simulink library "pmm"  (R2021b)
settings: Solver=VariableStepAuto  StartTime=0.0  StopTime=10.0  RelTol=1e-3
undefined symbols (not defined in the file): APMM_CoolgFanActCurr_X_pct, APMM_EWP1Curr_X_c, APMM_EWP3Curr_X_c, APMM_LVBattChktime_X_enum, APMM_LVBattChrgtime_X_enum, APMM_LVChrgLv_X_mV, ENUM_ANTITHEFT_ALARM, ENUM_ANTITHEFT_ARM, ENUM_ANTITHEFT_DISARM, ENUM_ANTITHEFT_WAIT, ENUM_APSSYSTEMSTA_REMOTEACTIVE, ENUM_CHRGPLUGSTA_NONE, ENUM_CRASHSTATE_FRONTFIRSTLV, ENUM_CRASHSTATE_LEFTSIDE, ENUM_CRASHSTATE_RIGHTSIDE, ENUM_DRIVETRAIN_AWD, ENUM_DRIVETRAIN_FWD, ENUM_DRIVETRAIN_RWD, ENUM_DRSEATSTA_EMPTY, ENUM_DRSEATSTA_INVALID, ENUM_DRSEATSTA_OCCUPIED, ENUM_EPBSTA_APPLIED, ENUM_GEARACTUALPOSN_D, ENUM_GEARACTUALPOSN_N, ENUM_GEARACTUALPOSN_P, ENUM_GEARACTUALPOSN_R, ENUM_HVBATTREADYPRE_READY, ENUM_OTACHKSTA_NOREQUEST, ENUM_OTACHKSTA_NOTIMEOUT, ENUM_OTACHKSTA_TIMEOUT, ENUM_PDKEYRAWLULOCK_INLOCK, ENUM_PDKEYRAWLULOCK_INUNLOCK, ENUM_PDKEYRAWPS_INPS, ENUM_PDKEYSTA_LOCK, ENUM_PDKEYSTA_PS, ENUM_PDKEYSTA_UNAVALIABLE, ENUM_PDKEYSTA_UNLOCK, ENUM_POWERSTA_OFF, ENUM_POWERSTA_OFFC, ENUM_POWERSTA_STANDBY, ENUM_PWRREQOTA_NOREQUEST, ENUM_PWRREQOTA_REQPOWEROFF, ENUM_PWRREQOTA_REQPOWERSTDBY, ENUM_PWRSTASW_READY, ENUM_V2LSTA_NOPLUG, ENUM_VEHICLETYPE_D31L24, ENUM_VEHMALFUNLEVEL_LEVEL3, ENUM_VEHMALFUNLEVEL_LEVEL4, FALSE, KPMM_AllDoorClosedHoldTime_s, KPMM_APSAllowThd_pct, KPMM_BattDownFailtime_s, KPMM_BattUpFailtime_s, KPMM_BattUpResetRty_cnt, KPMM_BattUpResetSW_flg, KPMM_BattUpResetTO_s, KPMM_BattUpRstDlyTO_s, KPMM_BrakeSWHoldTime_s, KPMM_CANValidChkFailtime_s, KPMM_ChrgPlugHoldTime_s ... (+87)
libraries: simulink x29, hcu_lib x24
(part 5 of 7)

== stateflow chart pmm/PMM/PMM/RequirementManagementForPowerUp ==
  state RequirementManagementForPowerUp
    note: [VINP_HVBattSOC_pct <= KPMM_HVBattSOCPwrDwnThd_pct]
    (default) -> (junction 135)
    RequirementManagementForPowerUp -> (junction 135) [order 2]
    (junction 135) -> (junction 3) : {VPMM_PwrUpReq_enum = ENUM_PWRUPREQ_NOREQUEST;
        |  VPMM_PwrStaSelect_enum = ENUM_PWRSTASELECT_NOREQUEST;}
    (junction 3) -> (junction 158) [order 1] : [(VPMM_PowerSta_enum == ENUM_POWERSTA_OFF || ...
        |   VPMM_PowerSta_enum == ENUM_POWERSTA_STANDBY) && ...
        |  VPMM_OTAPwrReqOFFChkSta_enum != ENUM_OTACHKSTA_NOTIMEOUT && ...
        |  VPMM_OTAPwrReqStdChkSta_enum != ENUM_OTACHKSTA_NOTIMEOUT]
    (junction 158) -> (junction 5) [order 1] : [(VPMM_DetectDoorOpened_flg || ...
        |   VPMM_BrkPedalRisingEdge_flg || ...
        |   (VPMM_BrkPedalPressed_flg && VPMM_PreOFF_flg)) && ...
        |  VPMM_PowerSta_enum == ENUM_POWERSTA_STANDBY]
        | {VPMM_PwrStaSelect_enum = ENUM_PWRSTASELECT_GOON;}
    (junction 3) -> (junction 6) [order 2]
    (junction 158) -> (junction 162) [order 2]
    (junction 5) -> (junction 8)
    (junction 8) -> (junction 167) [order 1] : [VPMM_PowerUpState_enum == ENUM_PUSTATE_POWERUPFAIL]
    (junction 8) -> (junction 169) [order 2] : {VPMM_PwrUpReq_enum = ENUM_PWRUPREQ_USERREQPU;}
    (junction 167) -> (junction 171)
    (junction 162) -> (junction 164) [order 1] : [(VPMM_ChrgPlugInRisingEdge_flg && VPMM_PowerSta_enum == ENUM_POWERSTA_STANDBY)|| ...
        |  (VPMM_LVSilentChrgReqStd_flg && ((!VINP_HoodSW_flg) || (VPMM_Delay4IVIWarnAct_flg))) || ...
        |  VPMM_LVSilentChrgReq_flg || ...
        |  (VINP_EvccAplusPwrUpReq_flg && VINP_ChrgPlugSta_enum != ENUM_CHRGPLUGSTA_NONE)]
        | {VPMM_PwrStaSelect_enum = ENUM_PWRSTASELECT_GOOFFC;}
    (junction 164) -> (junction 173) [order 1] : [VTQD_GearActualPosn_enum == ENUM_GEARACTUALPOSN_P && ...
        |  VINP_VehSpeed_kph < KPMM_PwrUpVehSpdThd_kph]
    (junction 162) -> (junction 237) [order 2]
    (junction 164) -> (junction 225) [order 2]
    (junction 173) -> (junction 239)
    (junction 237) -> (junction 239) [order 1] : [(VINP_PwrReq_OTA_enum == ENUM_PWRREQOTA_REQPOWERON && VINP_HVBattSOC_pct > KPMM_HVBattSOCPwrDwnThd_pct) || ...
        | (VINP_APSPwrReq_enum == ENUM_PWRREQPAPS_REQPWRREADY && VPMM_PwrReqRAPSAvail_flg)]
        | {VPMM_PwrStaSelect_enum = ENUM_PWRSTASELECT_GOON;}
    (junction 237) -> (junction 242) [order 2]
    (junction 239) -> (junction 244)
    (junction 242) -> (junction 244) [order 1] : [(VINP_SchedChgwake_flg == ENUM_SCHEDCHG_WAKE && ...
        |   VINP_ChrgPlugSta_enum != ENUM_CHRGPLUGSTA_NONE)]
        | {VPMM_PwrStaSelect_enum = ENUM_PWRSTASELECT_GOOFFC;}
    (junction 242) -> (junction 248) [order 2]
    (junction 244) -> (junction 250)
    (junction 248) -> (junction 250) [order 1] : [VINP_HVBPreheatPrecoolSta_enum == ENUM_HVBPRESTA_PREHEAT || ...
        |  VINP_HVBPreheatPrecoolSta_enum == ENUM_HVBPRESTA_PRECOOL]
        | {VPMM_PwrStaSelect_enum = ENUM_PWRSTASELECT_GOOFFA;}
    (junction 248) -> (junction 179) [order 2]
    (junction 250) -> (junction 194)
    (junction 179) -> (junction 181) [order 1] : [VINP_RePwrReqTbox_enum == ENUM_REPWRREQTBOX_REQVEHCHK || ...
        |  VINP_RePwrReqTbox_enum == ENUM_REPWRREQTBOX_REQDTC || ...
        |  VINP_RePwrReqTbox_enum == ENUM_REPWRREQTBOX_REQRADIO || ...
        |  VINP_RePwrReqTbox_enum == ENUM_REPWRREQTBOX_REQON || ...
        |  VINP_RePwrReqDKCT_enum == ENUM_REPWRREQDKC_REQVEHCHK || ...
        |  VINP_RePwrReqDKCT_enum == ENUM_REPWRREQDKC_REQDTC || ...
        |  VINP_RePwrReqDKCT_enum == ENUM_REPWRREQDKC_REQRADIO || ...
        |  VINP_RePwrReqDKCT_enum == ENUM_REPWRREQDKC_REQON]
        | {VPMM_PwrStaSelect_enum = ENUM_PWRSTASELECT_GOON;}
    (junction 179) -> (junction 183) [order 2]
    (junction 181) -> (junction 185)
    (junction 183) -> (junction 185) [order 1] : [VINP_RePwrReqTbox_enum == ENUM_REPWRREQTBOX_REQACTEMP || ...
        |  VINP_RePwrReqDKCT_enum == ENUM_REPWRREQDKC_REQACTEMP]
        | {VPMM_PwrStaSelect_enum = ENUM_PWRSTASELECT_GOOFFA;}
    (junction 183) -> (junction 190) [order 2]
    (junction 185) -> (junction 9)
    (junction 9) -> (junction 194) [order 1] : [VTQD_GearActualPosn_enum == ENUM_GEARACTUALPOSN_P && ...
        |  !VPMM_BMSWarn_flg && ...
        |  VINP_VehSpeed_kph < 2 && ...
        |  VINP_HVBattSOC_pct > KPMM_HVBattSOCPwrDwnThd_pct && ...
        |  VPMM_AllDoorClosed_flg && ...
        |  !VINP_HoodSW_flg && ...
        |  !VINP_TailgateSW_flg && ...
        |  VBCM_AntitheftSta_enum == ENUM_ANTITHEFT_ARM]
        | {VPMM_ReVehThdChkSta_enum = ENUM_REVEHSTA_CHECKOK;}
    (junction 194) -> (junction 197) [order 1] : [VPMM_PowerUpState_enum == ENUM_PUSTATE_POWERUPFAIL]
    (junction 9) -> (junction 11) [order 2]
    (junction 194) -> (junction 204) [order 2] : {VPMM_PwrUpReq_enum = ENUM_PWRUPREQ_SYSREQPU;}
    (junction 197) -> (junction 200)
    (junction 11) -> (junction 12) [order 1] : [VTQD_GearActualPosn_enum != ENUM_GEARACTUALPOSN_P]
        | {VPMM_ReVehThdChkSta_enum = ENUM_REVEHSTA_GEARPOSITIONERROR;}
    (junction 11) -> (junction 15) [order 2]
    (junction 15) -> (junction 16) [order 1] : [VPMM_BMSWarn_flg]
        | {VPMM_ReVehThdChkSta_enum = ENUM_REVEHSTA_HVBERR;}
    (junction 15) -> (junction 17) [order 2]
    (junction 17) -> (junction 18) [order 1] : [VINP_VehSpeed_kph >= 2]
        | {VPMM_ReVehThdChkSta_enum = ENUM_REVEHSTA_VEHNOTSTEADYSTATE;}
    (junction 17) -> (junction 21) [order 2]
    (junction 21) -> (junction 22) [order 1] : [VBCM_AntitheftSta_enum != ENUM_ANTITHEFT_ARM]
        | {VPMM_ReVehThdChkSta_enum = ENUM_REVEHSTA_ANTITHEFTNOTARM;}
    (junction 21) -> (junction 26) [order 2]
    (junction 26) -> (junction 27) [order 1] : [!VPMM_AllDoorClosed_flg || ...
        |  VINP_HoodSW_flg || ...
        |  VINP_TailgateSW_flg]
        | {VPMM_ReVehThdChkSta_enum = ENUM_REVEHSTA_ANYDOOROPEN;}
    (junction 26) -> (junction 29) [order 2]
    (junction 29) -> (junction 30) : {VPMM_ReVehThdChkSta_enum = ENUM_REVEHSTA_HVBSOCLOW;}
    (junction 29) -> (junction 31) [commented out] : {VPMM_ReVehThdChkSta_enum = ENUM_REVEHSTA_CHECKINVALID;}
    (junction 169) -> (junction 204)
    (junction 204) -> (junction 32)
    RequirementManagementForPowerUp -> (junction 32) [order 1] : [VPMM_PwrUpChk_flg]
        | {VPMM_PwrUpChk_flg = FALSE;}
    (junction 32) -> (junction 139) [order 1] : [VPMM_PowerUpState_enum == ENUM_PUSTATE_COMPLETED]
        | {VPMM_PwrUpChkFailtimer_s = 0;}
    (junction 32) -> (junction 141) [order 2]
    (junction 141) -> (junction 143) [order 1] : [VPMM_PwrUpChkFailtimer_s >= KPMM_PwrUpChkFailtime_s]
        | {VPMM_PwrUpChkFailtimer_s = 0;}
    (junction 141) -> (junction 145) [order 2] : {VPMM_PwrUpChk_flg = TRUE;
        |  VPMM_PwrUpChkFailtimer_s += task_time_s;}
  data: task_time_s input; VINP_HVBPreheatPrecoolSta_enum input; VINP_HVBattSOC_pct input; VINP_HoodSW_flg input; VINP_TailgateSW_flg input; VINP_SchedChgwake_flg input; VINP_VehSpeed_kph input; VPMM_AllDoorClosed_flg input; VBCM_AntitheftSta_enum input; VPMM_BMSWarn_flg input; VPMM_BrkPedalPressed_flg input; VPMM_BrkPedalRisingEdge_flg input; VPMM_ChrgPlugInRisingEdge_flg input; VPMM_DetectDoorOpened_flg input; VPMM_LVSilentChrgReq_flg input boolean; VPMM_PowerSta_enum input uint8; VTQD_GearActualPosn_enum input; VINP_PwrReq_OTA_enum input; VINP_RePwrReqDKCT_enum input; VINP_RePwrReqTbox_enum input; VPMM_PwrStaSelect_enum output; VPMM_PwrUpReq_enum output; VPMM_ReVehThdChkSta_enum output; ENUM_ANTITHEFT_ARM parameter; ENUM_GEARACTUALPOSN_P parameter; ENUM_HVBPRESTA_PRECOOL parameter; ENUM_HVBPRESTA_PREHEAT parameter; ENUM_POWERSTA_OFF parameter; ENUM_POWERSTA_STANDBY parameter; ENUM_PWRREQOTA_REQPOWERON parameter; ENUM_PWRSTASELECT_GOOFFA parameter; ENUM_PWRSTASELECT_GOOFFC parameter; ENUM_PWRSTASELECT_GOON parameter; ENUM_PWRSTASELECT_NOREQUEST parameter; ENUM_PWRUPREQ_NOREQUEST parameter; ENUM_PWRUPREQ_SYSREQPU parameter; ENUM_PWRUPREQ_USERREQPU parameter; ENUM_REPWRREQDKC_REQACTEMP parameter; ENUM_REPWRREQDKC_REQDTC parameter; ENUM_REPWRREQDKC_REQON parameter; ENUM_REPWRREQDKC_REQRADIO parameter; ENUM_REPWRREQDKC_REQVEHCHK parameter; ENUM_REPWRREQTBOX_REQACTEMP parameter; ENUM_REPWRREQTBOX_REQDTC parameter; ENUM_REPWRREQTBOX_REQON parameter; ENUM_REPWRREQTBOX_REQRADIO parameter; ENUM_REPWRREQTBOX_REQVEHCHK parameter; ENUM_REVEHSTA_ANTITHEFTNOTARM parameter; ENUM_REVEHSTA_ANYDOOROPEN parameter; ENUM_REVEHSTA_CHECKINVALID parameter; ENUM_REVEHSTA_CHECKOK parameter; ENUM_REVEHSTA_GEARPOSITIONERROR parameter; ENUM_REVEHSTA_HVBERR parameter; ENUM_REVEHSTA_HVBSOCLOW parameter; ENUM_REVEHSTA_VEHNOTSTEADYSTATE parameter; ENUM_SCHEDCHG_WAKE parameter; VPMM_PowerUpState_enum input uint8; VPMM_PwrUpChkFailtimer_s local single; VPMM_PwrUpChk_flg local boolean; ENUM_PUSTATE_COMPLETED parameter; FALSE parameter; TRUE parameter; VINP_ChrgPlugSta_enum input uint8; VINP_EvccAplusPwrUpReq_flg input boolean; VPMM_LVSilentChrgReqStd_flg input boolean; ENUM_PUSTATE_POWERUPFAIL parameter; VPMM_PreOFF_flg input boolean; ENUM_CHRGPLUGSTA_NONE parameter; VPMM_OTAPwrReqOFFChkSta_enum input uint8; VPMM_OTAPwrReqStdChkSta_enum input uint8; ENUM_OTACHKSTA_NOTIMEOUT parameter; KPMM_HVBattSOCPwrDwnThd_pct input; VINP_APSPwrReq_enum input uint8; VPMM_PwrReqRAPSAvail_flg input boolean; ENUM_PWRREQPAPS_REQPWRREADY parameter; KPMM_PwrUpChkFailtime_s input; VPMM_Delay4IVIWarnAct_flg input; KPMM_PwrUpVehSpdThd_kph input

== stateflow chart pmm/PMM/PMM/RequirementManagementForPowerStateConstrain ==
  state RequirementManagementForPowerStateConstrain
    (default) -> (junction 2) : {VPMM_TCountSta_enum = ENUM_TCOUNTSTA_NOCOUNTING;
        |  VPMM_PwrOffTimer_s = 0;}
    RequirementManagementForPowerStateConstrain -> (junction 2) [order 2]
    (junction 2) -> (junction 3) : {VPMM_PwrStaConstraint_enum = ENUM_PWRCONSTRAINT_NOREQUEST;}
    RequirementManagementForPowerStateConstrain -> (junction 3) [order 1] : [VPMM_ConstraintLoop_flg]
        | {VPMM_ConstraintLoop_flg = FALSE;}
    (junction 3) -> (junction 4) [order 1] : [VPMM_PowerSta_enum == ENUM_POWERSTA_ON || ...
        |  VPMM_PowerSta_enum == ENUM_POWERSTA_OFFA || ...
        |  VPMM_PowerSta_enum == ENUM_POWERSTA_OFFC]
    (junction 4) -> (junction 5) [order 1] : [VINP_PwrReq_OTA_enum == ENUM_PWRREQOTA_REQPOWERON || ...
        |  VINP_OFFACMODE_enum == ENUM_OFFACMODE_CAMP]
    (junction 3) -> (junction 6) [order 2]
    (junction 4) -> (junction 7) [order 2]
    (junction 5) -> (junction 8) : {VPMM_PwrStaConstraint_enum = ENUM_PWRCONSTRAINT_PWRSTAON;}
    (junction 7) -> (junction 8) [order 1] : [VINP_AVMOFFRecButt_flg == ENUM_AVMOFFRECBUTT_ON || ...
        |  VINP_OFFACMODE_enum == ENUM_OFFACMODE_PET || ...
        |  VINP_OFFACMODE_enum == ENUM_OFFACMODE_ON || ...
        |  VINP_HVBPreheatPrecoolSta_enum == ENUM_HVBPRESTA_PREHEAT || ...
        |  VINP_HVBPreheatPrecoolSta_enum == ENUM_HVBPRESTA_PRECOOL]
        | {VPMM_PwrStaConstraint_enum = ENUM_PWRCONSTRAINT_HVACTIVE;}
    (junction 7) -> (junction 80) [order 2]
    (junction 8) -> (junction 9) : {VPMM_TCountSta_enum = ENUM_TCOUNTSTA_NOCOUNTING;
        |  VPMM_PwrOffTimer_s = 0;
        |  VPMM_ConstraintLoop_flg = TRUE;}
    (junction 80) -> (junction 82) [order 1] : [VPMM_TCountSta_enum == ENUM_TCOUNTSTA_COUNTINGFINISH]
    (junction 82) -> (junction 90) [order 1] : [VPMM_PwrStaSW_enum == ENUM_PWRSTASW_PWRDOWN]
    (junction 80) -> (junction 10) [order 2]
    (junction 82) -> (junction 84) [order 2]
    (junction 90) -> (junction 92) : {VPMM_TCountSta_enum = ENUM_TCOUNTSTA_NOCOUNTING;}
    (junction 10) -> (junction 11) [order 1] : [(VPMM_PowerOffTSet_s > 0 && ...
        |   (VINP_RePwrReqTbox_enum == ENUM_REPWRREQTBOX_REQVEHCHK || ...
        |    VINP_RePwrReqTbox_enum == ENUM_REPWRREQTBOX_REQDTC || ...
        |    VINP_RePwrReqTbox_enum == ENUM_REPWRREQTBOX_REQRADIO || ...
        |    VINP_RePwrReqTbox_enum == ENUM_REPWRREQTBOX_REQON)) || ...
        |  (VPMM_PowerOffTSetDKC_enum > 0 && ...
        |   (VINP_RePwrReqDKCT_enum == ENUM_REPWRREQDKC_REQVEHCHK || ...
        |    VINP_RePwrReqDKCT_enum == ENUM_REPWRREQDKC_REQDTC || ...
        |    VINP_RePwrReqDKCT_enum == ENUM_REPWRREQDKC_REQRADIO || ...
        |    VINP_RePwrReqDKCT_enum == ENUM_REPWRREQDKC_REQON))]
    (junction 10) -> (junction 12) [order 2]
    (junction 11) -> (junction 13) : {VPMM_PwrStaConstraint_enum = ENUM_PWRCONSTRAINT_ONFORTIME;}
    (junction 12) -> (junction 13) [order 1] : [(VPMM_PowerOffTSet_s > 0 && ...
        |   VINP_RePwrReqTbox_enum == ENUM_REPWRREQTBOX_REQACTEMP) || ...
        |  (VPMM_PowerOffTSetDKC_enum > 0 && ...
        |   VINP_RePwrReqDKCT_enum == ENUM_REPWRREQDKC_REQACTEMP)]
        | {VPMM_PwrStaConstraint_enum = ENUM_PWRCONSTRAINT_HVFORTIME;}
    (junction 13) -> (junction 14) [order 1] : [(VPMM_PowerOffTSet_s >= VPMM_PowerOffTSetDKC_enum && VPMM_PwrOffTimer_s >= VPMM_PowerOffTSet_s) || ...
        |  (VPMM_PowerOffTSetDKC_enum > VPMM_PowerOffTSet_s && VPMM_PwrOffTimer_s >= VPMM_PowerOffTSetDKC_enum)]
    (junction 12) -> (junction 15) [order 2] : {VPMM_TCountSta_enum = ENUM_TCOUNTSTA_NOCOUNTING;
        |  VPMM_PwrOffTimer_s = 0;}
    (junction 13) -> (junction 16) [order 2] : {VPMM_TCountSta_enum = ENUM_TCOUNTSTA_TIMMERCOUNTING;
        |  VPMM_PwrOffTimer_s += task_time_s;
        |  VPMM_ConstraintLoop_flg = TRUE;}
    (junction 14) -> (junction 17) : {VPMM_TCountSta_enum = ENUM_TCOUNTSTA_COUNTINGFINISH;
        |  VPMM_PwrStaConstraint_enum = ENUM_PWRCONSTRAINT_NOREQUEST;
        |  VPMM_PwrOffTimer_s = 0;}
  data: task_time_s input; VPMM_PowerSta_enum input; VINP_AVMOFFRecButt_flg input; VINP_HVBPreheatPrecoolSta_enum input; VINP_OFFACMODE_enum input; VPMM_PowerOffTSet_s input; VPMM_PowerOffTSetDKC_enum input; VINP_PwrReq_OTA_enum input; VINP_RePwrReqDKCT_enum input; VINP_RePwrReqTbox_enum input; VPMM_PwrStaConstraint_enum output; VPMM_TCountSta_enum output; VPMM_PwrOffTimer_s local single; ENUM_AVMOFFRECBUTT_ON parameter; ENUM_HVBPRESTA_PRECOOL parameter; ENUM_HVBPRESTA_PREHEAT parameter; ENUM_OFFACMODE_CAMP parameter; ENUM_OFFACMODE_ON parameter; ENUM_OFFACMODE_PET parameter; ENUM_POWERSTA_OFFA parameter; ENUM_POWERSTA_OFFC parameter; ENUM_POWERSTA_ON parameter; ENUM_PWRCONSTRAINT_HVACTIVE parameter; ENUM_PWRCONSTRAINT_HVFORTIME parameter; ENUM_PWRCONSTRAINT_NOREQUEST parameter; ENUM_PWRCONSTRAINT_ONFORTIME parameter; ENUM_PWRCONSTRAINT_PWRSTAON parameter; ENUM_PWRREQOTA_REQPOWERON parameter; ENUM_REPWRREQDKC_REQACTEMP parameter; ENUM_REPWRREQDKC_REQDTC parameter; ENUM_REPWRREQDKC_REQON parameter; ENUM_REPWRREQDKC_REQRADIO parameter; ENUM_REPWRREQDKC_REQVEHCHK parameter; ENUM_REPWRREQTBOX_REQACTEMP parameter; ENUM_REPWRREQTBOX_REQDTC parameter; ENUM_REPWRREQTBOX_REQON parameter; ENUM_REPWRREQTBOX_REQRADIO parameter; ENUM_REPWRREQTBOX_REQVEHCHK parameter; ENUM_TCOUNTSTA_COUNTINGFINISH parameter; ENUM_TCOUNTSTA_NOCOUNTING parameter; ENUM_TCOUNTSTA_TIMMERCOUNTING parameter; VPMM_ConstraintLoop_flg local boolean; FALSE parameter; TRUE parameter; VPMM_PwrStaSW_enum input; ENUM_PWRSTASW_PWRDOWN parameter
